simulink model "onlyProportional"  (R2024b)
settings: Solver=VariableStepAuto  StartTime=0.0  StopTime=15  FixedStep=0.001  RelTol=1e-3
InitFcn:
  | LCS_parameters
undefined symbols (not defined in the file or in its folder): a0, a1, a2, a3, a4, gearRatio
libraries: simulink x2, Solver_SF x1
settings Model: Creator=account  LastModifiedBy=xoxi.1

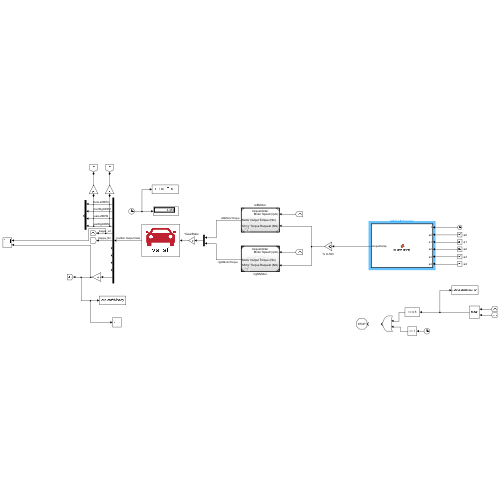
[thumbnail: Simulink's stored preview of the top-level diagram]
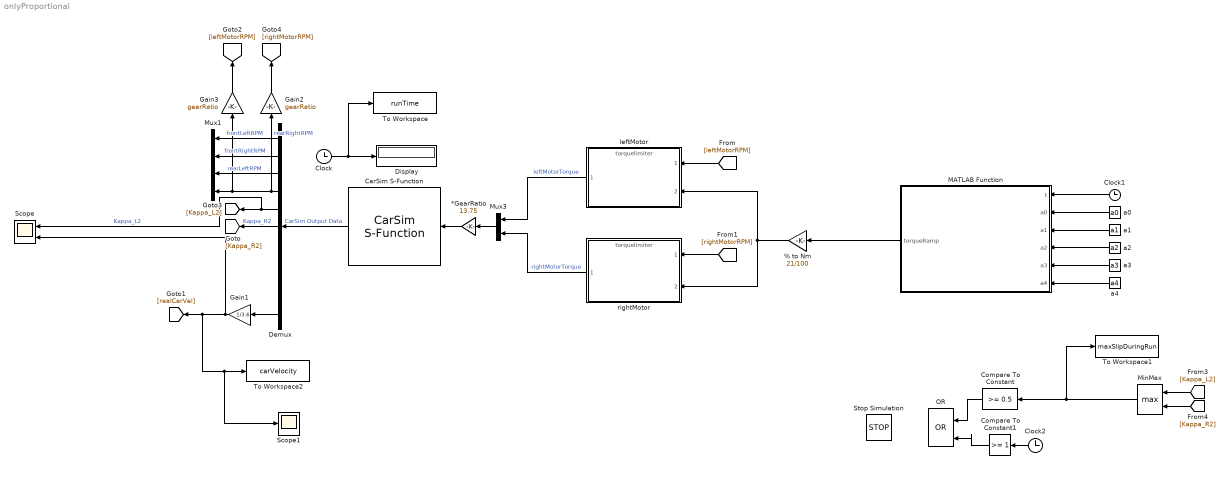
== system onlyProportional ==
  % to Nm : Gain  Gain=21/100
  *GearRatio : Gain  Gain=13.75
  CarSim S-Function : Solver_SF/CarSim S-Function  Priority=1  SIMFILE=simfile.sim  Run_RTs=off  vs_state_ind=Run  StopMode_ind=Vehicle Model
  Clock : Clock
  Clock1 : Clock
  Clock2 : Clock
  Compare To Constant : simulink/Logic and Bit Operations/Compare To Constant  relop=>=  const=0.5  OutDataTypeStr=boolean
  Compare To Constant1 : simulink/Logic and Bit Operations/Compare To Constant  relop=>=  const=1  OutDataTypeStr=boolean
  Demux : Demux  Outputs=11
  Display : Display
  Gain1 : Gain  Gain=1/3.6
  Gain2 : Gain  Gain=gearRatio
  Gain3 : Gain  Gain=gearRatio
  MATLAB Function : MATLAB Function  TreatAsAtomicUnit=on
  MinMax : MinMax  Function=max  Inputs=2
  Mux1 : Mux
  Mux3 : Mux  Inputs=2
  OR : Logic  Operator=OR  IconShape=distinctive  AllPortsSameDT=off  OutDataTypeStr=boolean
  Scope : Scope  NumInputPorts=2
  Scope1 : Scope
  Stop Simulation : Stop
  To Workspace : ToWorkspace  VariableName=runTime  SaveFormat=Timeseries  SampleTime=-1
      settings: Save2DSignal=2-D array (concatenate along first dimension)
  To Workspace1 : ToWorkspace  VariableName=maxSlipDuringRun  SampleTime=-1
      settings: Save2DSignal=2-D array (concatenate along first dimension)
  To Workspace2 : ToWorkspace  VariableName=carVelocity  SampleTime=-1
      settings: Save2DSignal=2-D array (concatenate along first dimension)
  a0 : Constant  Value=a0
  a1 : Constant  Value=a1
  a2 : Constant  Value=a2
  a3 : Constant  Value=a3
  a4 : Constant  Value=a4
  leftMotor : ModelReference  ModelNameDialog=torquelimiter.slx  SimulationMode=Normal  ModelReferenceVersion=1.5
  rightMotor : ModelReference  ModelNameDialog=torquelimiter.slx  SimulationMode=Normal  ModelReferenceVersion=1.5
  wires:
  CarSim S-Function/1 -> Demux/1  "CarSim Output Data"
  Demux/1 -> Mux1/1  "frontLeftRPM"
  Demux/2 -> Mux1/2  "frontRightRPM"
  Demux/3 -> Mux1/3  "rearLeftRPM"
  Clock/1 -> To Workspace/1, Display/1
  leftMotor/1 -> Mux3/1  "leftMotorTorque"
  rightMotor/1 -> Mux3/2  "rightMotorTorque"
  Demux/4 -> Mux1/4, Gain3/1, Gain2/1  "rearRightRPM"
  [rightMotorRPM] -> rightMotor/1
  [leftMotorRPM] -> leftMotor/1
  Demux/5 -> Scope/1, [Kappa_L2]  "Kappa_L2"
  Demux/6 -> [Kappa_R2]  "Kappa_R2"
  % to Nm/1 -> rightMotor/2, leftMotor/2
  *GearRatio/1 -> CarSim S-Function/1
  Mux3/1 -> *GearRatio/1
  Gain3/1 -> [leftMotorRPM]
  Gain2/1 -> [rightMotorRPM]
  Demux/11 -> Gain1/1
  Gain1/1 -> Scope/2, Scope1/1, To Workspace2/1, [realCarVel]
  MinMax/1 -> To Workspace1/1, Compare To Constant/1
  [Kappa_L2] -> MinMax/1
  [Kappa_R2] -> MinMax/2
  Compare To Constant1/1 -> OR/2
  Clock2/1 -> Compare To Constant1/1
  MATLAB Function/1(torqueRamp) -> % to Nm/1
  Clock1/1 -> MATLAB Function/1(t)
  a4/1 -> MATLAB Function/6(a4)
  a3/1 -> MATLAB Function/5(a3)
  a2/1 -> MATLAB Function/4(a2)
  a1/1 -> MATLAB Function/3(a1)
  a0/1 -> MATLAB Function/2(a0)
  Compare To Constant/1 -> OR/1

== matlab function onlyProportional/MATLAB Function ==
  data: t input; a0 input; torqueRamp output; a1 input; a2 input; a3 input; a4 input
function torqueRamp = launchRamp(t, a0, a1, a2, a3, a4)
    % T(t) = a4*t^4 + a3*t^3 + a2*t^2 + a1*t + a0
if t <= 1.0
        torqueRamp = a4*t^4 + a3*t^3 + a2*t^2 + a1*t + a0;
else
        torqueRamp = a4 + a3 + a2 + a1 + a0;  % holds T(1) value
end
% Clamp to 0-100%
    torqueRamp = min(max(torqueRamp, 0), 100);
end
